simulink model "Model1_2019b"  (R2019b)
settings: Solver=ode4  StartTime=0.0  StopTime=10  FixedStep=0.01  RelTol=1e-3
values from neighbouring files (symbols this model uses):
  A = [0 1 0;     0 -0.875 -20;     0 0 -50]    [Zadanie1.m]    (also in Zadanie2.m = [0 1 0 0;     0 -1 0 0;     0 0 0 1;     0 0 0 -1])
  B = [0;      0;      50]    [Zadanie1.m]    (also in Zadanie2.m = [0 0;     1 0;     0 0;     0 1])
  K = -Km    [Zadanie1.m]
settings Model: Creator=grzyb  LastModifiedBy=SARIS

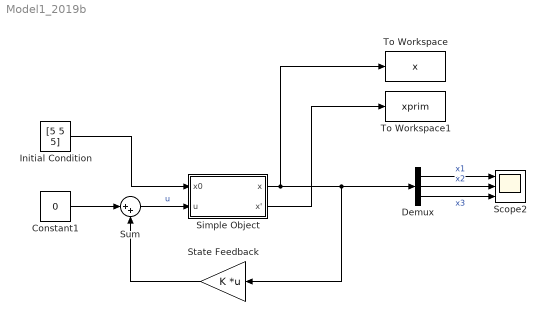
== system Model1_2019b ==
  Constant1 : Constant  Value=0
  Demux : Demux  Outputs=3
  Initial Condition : Constant  Value=[5 5 5]
  Scope2 : Scope  NumInputPorts=3
  Simple Object : Subsystem
  State Feedback : Gain  Gain=K  Multiplication=Matrix(K*u)
  Sum : Sum  Inputs=|++
  To Workspace : ToWorkspace  VariableName=x  SampleTime=-1
  To Workspace1 : ToWorkspace  VariableName=xprim  SampleTime=-1
  wires:
  Simple Object/1(x) -> Demux/1, State Feedback/1, To Workspace/1
  Initial Condition/1 -> Simple Object/1(x0)
  Sum/1 -> Simple Object/2(u)  "u"
  State Feedback/1 -> Sum/2
  Constant1/1 -> Sum/1
  Demux/1 -> Scope2/1  "x1"
  Demux/2 -> Scope2/2  "x2"
  Demux/3 -> Scope2/3  "x3"
  Simple Object/2(x') -> To Workspace1/1

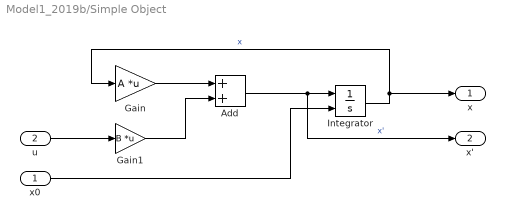
== system Model1_2019b/Simple Object ==
  x0 : Inport
  u : Inport  Port=2
  Add : Sum
  Gain : Gain  Gain=A  Multiplication=Matrix(K*u)
  Gain1 : Gain  Gain=B  Multiplication=Matrix(K*u)
  Integrator : Integrator  InitialConditionSource=external
  x : Outport
  x' : Outport  Port=2
  wires:
  Integrator/1 -> x/1, Gain/1  "x"
  Add/1 -> x'/1, Integrator/1  "x'"
  Gain/1 -> Add/1
  Gain1/1 -> Add/2
  u/1 -> Gain1/1
  x0/1 -> Integrator/2
